simulink model "simulink_model"  (R2025a)
settings: Solver=VariableStepAuto  StartTime=0.0  StopTime=2  FixedStep=1e-4  RelTol=1e-2  AbsTol=1e-5
values from neighbouring files (symbols this model uses):
  beta = Nf/(1+Nf)    [controller.m]
  CF = 80    [main.m]    (also in speed_control.m = 200)
  CPR = 14    [main.m]
  Kd = 1/p * Kp + 1/(Z1*Z2)    [controller.m]    (also in main.m = K_out.Kd)
  Ki = K_out.Ki    [main.m]    (also in speed_control.m = 1   * K0; test.m = 1)
  Kjt = 1/n2 * 1/n1    [main.m]
  Kp = 1/p - (Z1+Z2) / (Z1*Z2)    [controller.m]    (also in main.m = K_out.Kp; speed_control.m = -1/z * K0; test.m = 0.125)
  Ktj = 1/Kjt    [main.m]
  nKm = Km    [main.m]
  PWM_freq = 20 * 1e3    (= 20000)    [controller.m]    (also in speed_control.m = 10000)
  Vmotor = 12    [main.m]
  yd = 0.02    [main.m]
  Ye = 1/(s*Lw + Rw)    [main.m]
  Ym = Ztot    [main.m]
libraries: dspsigops x3, simulink_extras x2, simulink x1
settings Model: Creator=flipa  LastModifiedBy=flipa

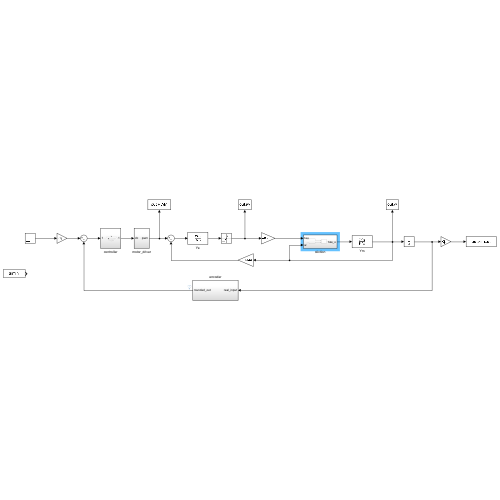
[thumbnail: Simulink's stored preview of the top-level diagram]
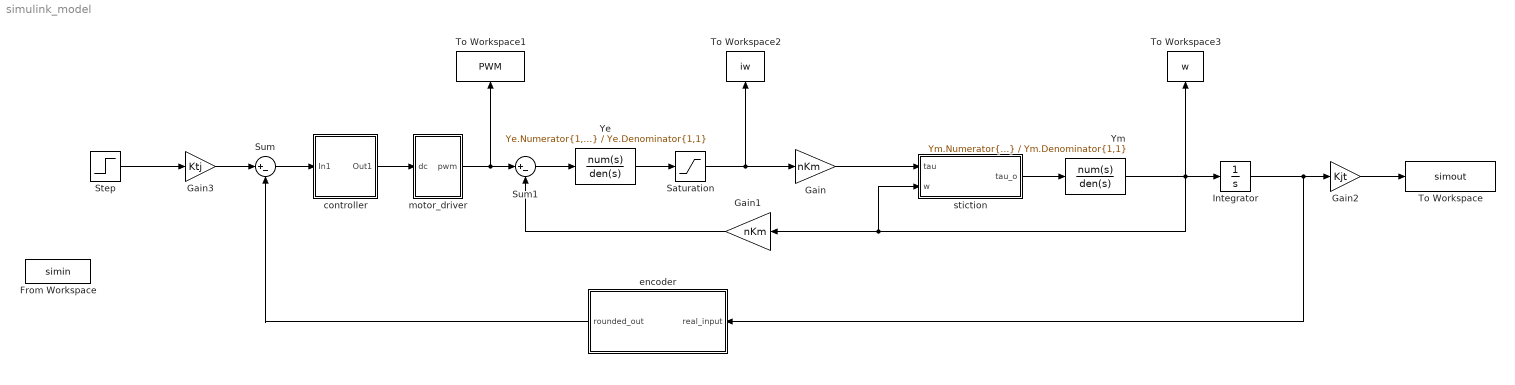
== system simulink_model ==
  From Workspace : FromWorkspace  VariableName=simin
  Gain : Gain  Gain=nKm
  Gain1 : Gain  Gain=nKm
  Gain2 : Gain  Gain=Kjt
  Gain3 : Gain  Gain=Ktj
  Integrator : Integrator
  Saturation : Saturate  UpperLimit=1.5  LowerLimit=-1.5
  Step : Step  Time=0  After=yd  SampleTime=0
  Sum : Sum  Inputs=|+-
  Sum1 : Sum  Inputs=|+-
  To Workspace : ToWorkspace  VariableName=simout  SaveFormat=Timeseries  SampleTime=-1
  To Workspace1 : ToWorkspace  VariableName=PWM  SaveFormat=Timeseries  SampleTime=-1
  To Workspace2 : ToWorkspace  VariableName=iw  SaveFormat=Timeseries  SampleTime=-1
  To Workspace3 : ToWorkspace  VariableName=w  SaveFormat=Timeseries  SampleTime=-1
  Ye : TransferFcn  Numerator=Ye.Numerator{1,1}  Denominator=Ye.Denominator{1,1}  ContinuousStateAttributes='iw'
  Ym : TransferFcn  Numerator=Ym.Numerator{1,1}  Denominator=Ym.Denominator{1,1}  ContinuousStateAttributes='iw'
  controller : Subsystem
  encoder : Subsystem
  motor_driver : Subsystem
  stiction : Subsystem
  wires:
  Gain/1 -> stiction/1(tau)
  Gain1/1 -> Sum1/2
  Sum1/1 -> Ye/1
  Gain2/1 -> To Workspace/1
  Step/1 -> Gain3/1
  Gain3/1 -> Sum/1
  motor_driver/1(pwm) -> To Workspace1/1, Sum1/1
  Sum/1 -> controller/1(In1)
  controller/1(Out1) -> motor_driver/1(dc)
  Ye/1 -> Saturation/1
  Integrator/1 -> encoder/1(real_input), Gain2/1
  encoder/1(rounded_out) -> Sum/2
  Saturation/1 -> To Workspace2/1, Gain/1
  stiction/1(tau_o) -> Ym/1
  Ym/1 -> To Workspace3/1, Integrator/1, stiction/2(w), Gain1/1

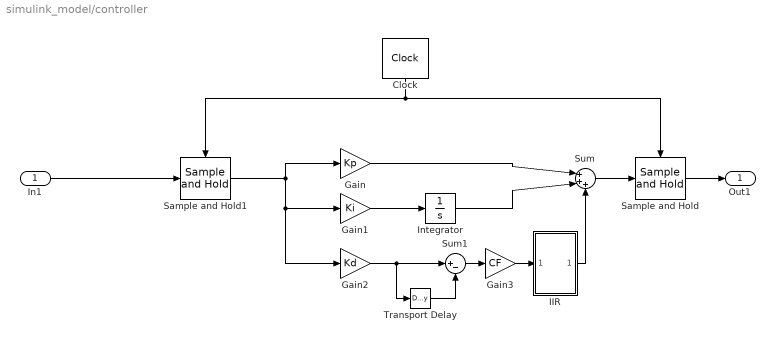
== system simulink_model/controller ==
  In1 : Inport
  Clock : simulink_extras/Flip Flops/Clock  period=1/CF
  Gain : Gain  Gain=Kp
  Gain1 : Gain  Gain=Ki
  Gain2 : Gain  Gain=Kd
  Gain3 : Gain  Gain=CF
  IIR : Subsystem
  Integrator : Integrator
  Sample and Hold : dspsigops/Sample and Hold  trig=Rising edge  initCond=0  latchinput=off
  Sample and Hold1 : dspsigops/Sample and Hold  trig=Rising edge  initCond=0  latchinput=off
  Sum : Sum  Inputs=|+++
  Sum1 : Sum  Inputs=|+-
  Transport Delay : TransportDelay  DelayTime=1/CF
  Out1 : Outport
  wires:
  In1/1 -> Sample and Hold1/1
  Sum/1 -> Sample and Hold/1
  Sample and Hold/1 -> Out1/1
  Clock/1 -> Sample and Hold/Trigger, Sample and Hold1/Trigger
  Gain1/1 -> Integrator/1
  Integrator/1 -> Sum/2
  Gain/1 -> Sum/1
  Sample and Hold1/1 -> Gain2/1, Gain1/1, Gain/1
  Transport Delay/1 -> Sum1/2
  Gain2/1 -> Sum1/1, Transport Delay/1
  Sum1/1 -> Gain3/1
  Gain3/1 -> IIR/1(In1)
  IIR/1(Out1) -> Sum/3

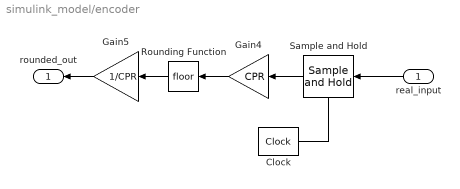
== system simulink_model/encoder ==
  real_input : Inport
  Clock : simulink_extras/Flip Flops/Clock  period=T_encoder
  Gain4 : Gain  Gain=CPR
  Gain5 : Gain  Gain=1/CPR
  Rounding Function : Rounding
  Sample and Hold : dspsigops/Sample and Hold  trig=Rising edge  initCond=0  latchinput=off
  rounded_out : Outport
  wires:
  Gain4/1 -> Rounding Function/1
  Rounding Function/1 -> Gain5/1
  Gain5/1 -> rounded_out/1
  Sample and Hold/1 -> Gain4/1
  Clock/1 -> Sample and Hold/Trigger
  real_input/1 -> Sample and Hold/1

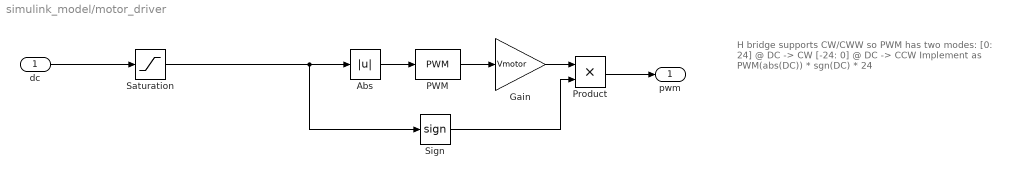
== system simulink_model/motor_driver ==
  note: H bridge supports CW/CWW so PWM has two modes:
      |
      | [0: 24] @ DC -> CW
      | [-24: 0] @ DC -> CCW
      |
      | Implement as
      | PWM(abs(DC)) * sgn(DC) * 24
  dc : Inport
  Abs : Abs  SaturateOnIntegerOverflow=off
  Gain : Gain  Gain=Vmotor
  PWM : simulink/Discontinuities/PWM  DisableCoverage=on  Period=1/PWM_freq  InitialDelay=0  DisallowZeroDutyCycle=off  RunAtFixedTimeIntervals=off  SampleTime=0.1
  Product : Product
  Saturation : Saturate  UpperLimit=1  LowerLimit=-1
  Sign : Signum
  pwm : Outport
  wires:
  PWM/1 -> Gain/1
  dc/1 -> Saturation/1
  Gain/1 -> Product/1
  Abs/1 -> PWM/1
  Product/1 -> pwm/1
  Sign/1 -> Product/2
  Saturation/1 -> Sign/1, Abs/1

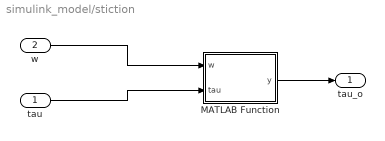
== system simulink_model/stiction ==
  tau : Inport
  w : Inport  Port=2
  MATLAB Function : MATLAB Function  TreatAsAtomicUnit=on
  tau_o : Outport
  wires:
  tau/1 -> MATLAB Function/2(tau)
  MATLAB Function/1(y) -> tau_o/1
  w/1 -> MATLAB Function/1(w)

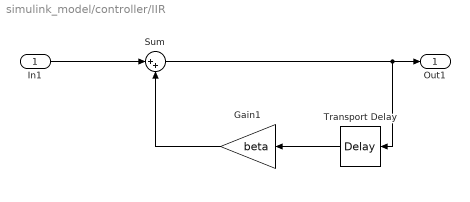
== system simulink_model/controller/IIR ==
  In1 : Inport
  Gain1 : Gain  Gain=beta
  Sum : Sum  Inputs=|++
  Transport Delay : TransportDelay  DelayTime=1/CF
  Out1 : Outport
  wires:
  In1/1 -> Sum/1
  Sum/1 -> Transport Delay/1, Out1/1
  Transport Delay/1 -> Gain1/1
  Gain1/1 -> Sum/2

== matlab function simulink_model/stiction/MATLAB Function ==
  data: w input; y output; tau input
function y = fcn(w, tau)
    
    Rw = 8;
    Km = 0.0180;
    Vbreak = 3;     % Voltage at which we can overcome static friction 
    Ibreak = Vbreak / Rw;

    tau0 = Km * Ibreak;
    
    % Applied torque must overcome static friction when speed is 0 
    stuck = (w == 0) & (abs(tau) < tau0);

    if stuck
        y = 0;
    else
        y = tau - tau0 * 0.5;
    end
